simulink model "Unicycle_AVF"  (R2024a)
settings: Solver=VariableStepAuto  StartTime=0.0  StopTime=500  FixedStep=0.1  MaxStep=0.1  RelTol=1e-3
settings Model: Creator=qiaoyike  LastModifiedBy=qiaoyike
settings RTWCC: GPUComputeCapability=3.5

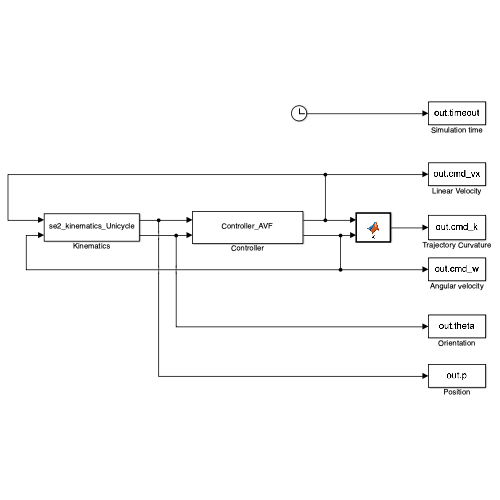
[thumbnail: Simulink's stored preview of the top-level diagram]
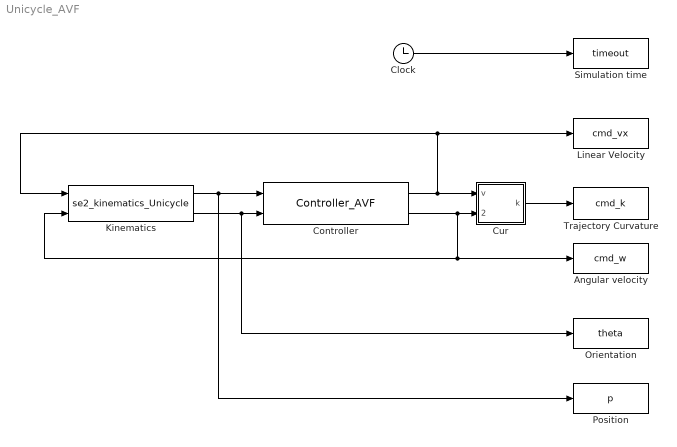
== system Unicycle_AVF ==
  Angular velocity : ToWorkspace  VariableName=cmd_w  SampleTime=-1
  Clock : Clock
  Controller : M-S-Function  FunctionName=Controller_AVF  Parameters=pd,theta_d  mask{pd=[-8;9.79717439317883e-16], theta_d=4.71238898038469}
      mask prompts: pd "Desired posistion [xd;yd]"; theta_d "Desired orientaion in S"
      mask DialogControl ParameterGroupVar Prompt: 参数
  Cur : MATLAB Function  TreatAsAtomicUnit=on
  Kinematics : M-S-Function  FunctionName=se2_kinematics_Unicycle  Parameters=p0,theta0  mask{p0=[8.59229469246884;12.6765706716381], theta0=5.00981357947841}
      mask prompts: p0 "Initial position [x0; y0]"; theta0 "Initial attitude theta0"
      mask DialogControl ParameterGroupVar Prompt: 参数
  Linear Velocity : ToWorkspace  VariableName=cmd_vx  SampleTime=-1
  Orientation : ToWorkspace  VariableName=theta  SampleTime=-1
  Position : ToWorkspace  VariableName=p  SampleTime=-1
  Simulation time : ToWorkspace  VariableName=timeout  SampleTime=-1
  Trajectory Curvature : ToWorkspace  VariableName=cmd_k  SampleTime=-1
  wires:
  Clock/1 -> Simulation time/1
  Kinematics/1 -> Controller/1, Position/1
  Kinematics/2 -> Controller/2, Orientation/1
  Controller/1 -> Kinematics/1, Linear Velocity/1, Cur/1(v)
  Controller/2 -> Kinematics/2, Angular velocity/1, Cur/2(Omega)
  Cur/1(k) -> Trajectory Curvature/1

== matlab function Unicycle_AVF/Cur ==
  data: v input; k output; Omega input
function k = k(v,Omega)
k = norm(Omega)/norm(v);
